simulink model "test_torque"  (R2024b)
settings: Solver=FixedStepDiscrete  StartTime=0.0  StopTime=inf  FixedStep=0.001  RelTol=1e-3
values from neighbouring files (symbols this model uses):
  test_torque_max_nm = 20.0    [test_torque.sldd]
libraries: speedgoatlib_IO614 x4, canmsglib x2
settings Model: DataDictionary=test_torque.sldd  Creator=MFE-HPC  LastModifiedBy=MFE-HPC
settings SolverCC: ConcurrentTasks=on  PositivePriorityOrder=on
settings OptimizationCC: BlockReduction=off  OptimizeBlockIOStorage=off
settings DebuggingCC: TasksWithSamePriorityMsg=none
settings HardwareCC: ProdBitPerLong=64  ProdLongLongMode=on  ProdHWDeviceType=Intel->x86-64 (Linux 64)
settings RTWCC: Description=Speedgoat Real-Time Target Machine  SystemTargetFile=speedgoat.tlc  TemplateMakefile=slrealtime_default_tmf  Toolchain=Simulink Real-Time Toolchain  BuildConfiguration=Faster Runs  CodeExecutionProfiling=on  TargetLang=C++
settings SimulinkRealTimeTargetCC: InstructionSetFMA=off  LogToMDFFile=off

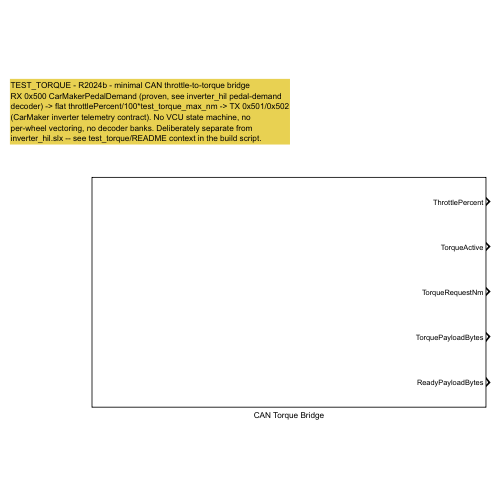
[thumbnail: Simulink's stored preview of the top-level diagram]
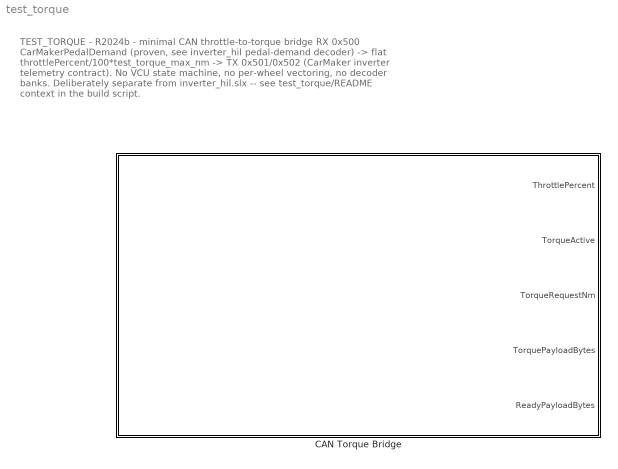
== system test_torque ==
  note: TEST_TORQUE - R2024b - minimal CAN throttle-to-torque bridge
      | RX 0x500 CarMakerPedalDemand (proven, see inverter_hil pedal-demand
      | decoder) -> flat throttlePercent/100*test_torque_max_nm -> TX 0x501/0x502
      | (CarMaker inverter telemetry contract). No VCU state machine, no
      | per-wheel vectoring, no decoder banks. Deliberately separate from
      | inverter_hil.slx -- see test_torque/README context in the build script.
  CAN Torque Bridge : Subsystem

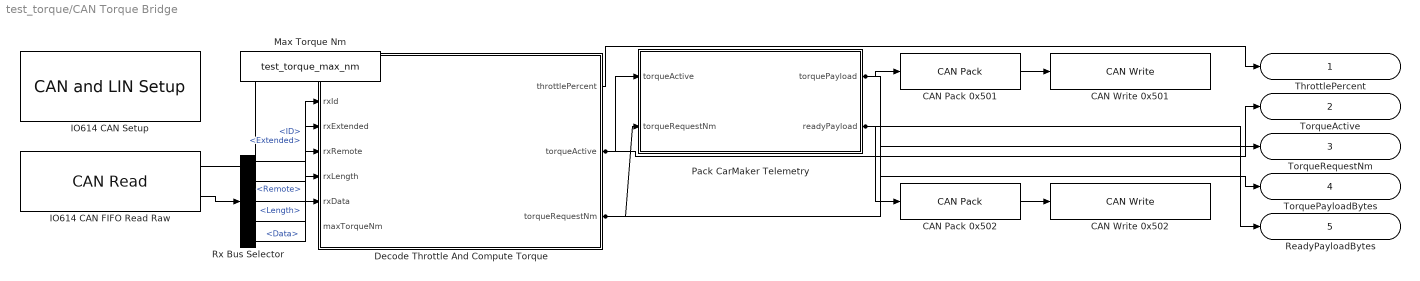
== system test_torque/CAN Torque Bridge ==
  CAN Pack 0x501 : canmsglib/CAN Pack  Description=Torque payload, CarMaker inverter telemetry ID 0x501  MsgList=(none)  MsgName=CAN Msg  MsgIDType=Standard (11-bit identifier)  MsgIdentifier=1281  CANIDInput=off  MsgLength=8  Remote=off  ApplyMinMax=off  BusOutput=off  SignalInfo={}
      settings: LibrarySourceBlock=canlib/CAN Pack  DataFormat=raw data
  CAN Pack 0x502 : canmsglib/CAN Pack  Description=Ready payload, CarMaker inverter telemetry ID 0x502  MsgList=(none)  MsgName=CAN Msg  MsgIDType=Standard (11-bit identifier)  MsgIdentifier=1282  CANIDInput=off  MsgLength=8  Remote=off  ApplyMinMax=off  BusOutput=off  SignalInfo={}
      settings: LibrarySourceBlock=canlib/CAN Pack  DataFormat=raw data
  CAN Write 0x501 : speedgoatlib_IO614/CAN Write   Description=Transmits CarMaker telemetry ID 0x501  moduleType=IO614  id=1  channel=1  canType=CAN (HS)  useBusIn=off  numOfMsg=1  enableInput=off  enableStatusPort=on  initValues=[614 1 0.001 0 1 1 1 1 0 0]  ts=0.001
  CAN Write 0x502 : speedgoatlib_IO614/CAN Write   Description=Transmits CarMaker telemetry ID 0x502  moduleType=IO614  id=1  channel=1  canType=CAN (HS)  useBusIn=off  numOfMsg=1  enableInput=off  enableStatusPort=on  initValues=[614 1 0.001 0 1 1 1 1 0 0]  ts=0.001
  Decode Throttle And Compute Torque : MATLAB Function  TreatAsAtomicUnit=on
  IO614 CAN FIFO Read Raw : speedgoatlib_IO614/CAN Read   moduleType=IO614  id=1  channel=1  canType=CAN (HS)  useBusOut=on  HasMulRead=Single Read from Buffer (FIFO)  MsgIDlist=[1 2]  isEFF=off  LabelInHex=on  enableInput=off  ts=0.001  initValues=[614 1 0.001 0 1 1 0 1 0 1 2 1 2]
  IO614 CAN Setup : speedgoatlib_IO614/CAN and LIN Setup   moduleInitValues="[614    1    1   -1   -1]"  id=1  moduleType=IO614  pciSlot=-1  canChn1=CAN (HS)  canChn2=Disabled  canChn3=Disabled  canChn4=Disabled  linChn1=Disabled  linChn2=Disabled  canInitStructArray=[]  canTermStructArray=[]  canChn1InitValues="[2   2   1  31   8   2   1   5   2]"  arbBdrChn1=1.0 MBaud  arbManBdrChn1=[2,1,31,8]  fdBdrChn1=5.0 MBaud  fdManBdrChn1=[2,1,5,2]  canChn2InitValues="[1   2   1  31   8   2   1   5   2]"  arbBdrChn2=1.0 MBaud  arbManBdrChn2=[2,1,31,8]  fdBdrChn2=5.0 MBaud  fdManBdrChn2=[2,1,5,2]  canChn3InitValues="[1   2   1  31   8   2   1   5   2]"  arbBdrChn3=1.0 MBaud  arbManBdrChn3=[2,1,31,8]  fdBdrChn3=5.0 MBaud  fdManBdrChn3=[2,1,5,2]  canChn4InitValues="[1   2   1  31   8   2   1   5   2]"  arbBdrChn4=1.0 MBaud  arbManBdrChn4=[2,1,31,8]  fdBdrChn4=5.0 MBaud  fdManBdrChn4=[2,1,5,2]  bdrLIN1=19200  linChn1InitValues="[1  19200]"  bdrLIN2=19200  linChn2InitValues="[1  19200]"
      settings: LibrarySourceBlock=speedgoatlib_CANLIN_OfA2/CAN and LIN Setup
  Max Torque Nm : Constant  Value=test_torque_max_nm  SampleTime=0.001
  Pack CarMaker Telemetry : MATLAB Function  TreatAsAtomicUnit=on
  Rx Bus Selector : BusSelector  OutputSignals=ID,Extended,Remote,Length,Data
  ThrottlePercent : Outport
  TorqueActive : Outport  Port=2
  TorqueRequestNm : Outport  Port=3
  TorquePayloadBytes : Outport  Port=4
  ReadyPayloadBytes : Outport  Port=5
  wires:
  ? -> ?
  IO614 CAN FIFO Read Raw/2 -> Rx Bus Selector/1
  IO614 CAN FIFO Read Raw/1 -> Decode Throttle And Compute Torque/1(rxDataPresent)
  Rx Bus Selector/1 -> Decode Throttle And Compute Torque/2(rxId)  "<ID>"
  Rx Bus Selector/2 -> Decode Throttle And Compute Torque/3(rxExtended)  "<Extended>"
  Rx Bus Selector/3 -> Decode Throttle And Compute Torque/4(rxRemote)  "<Remote>"
  Rx Bus Selector/4 -> Decode Throttle And Compute Torque/5(rxLength)  "<Length>"
  Rx Bus Selector/5 -> Decode Throttle And Compute Torque/6(rxData)  "<Data>"
  Max Torque Nm/1 -> Decode Throttle And Compute Torque/7(maxTorqueNm)
  Decode Throttle And Compute Torque/2(torqueActive) -> Pack CarMaker Telemetry/1(torqueActive), TorqueActive/1
  Decode Throttle And Compute Torque/3(torqueRequestNm) -> Pack CarMaker Telemetry/2(torqueRequestNm), TorqueRequestNm/1
  Pack CarMaker Telemetry/1(torquePayload) -> CAN Pack 0x501/1, TorquePayloadBytes/1
  CAN Pack 0x501/1 -> CAN Write 0x501/1
  Pack CarMaker Telemetry/2(readyPayload) -> CAN Pack 0x502/1, ReadyPayloadBytes/1
  CAN Pack 0x502/1 -> CAN Write 0x502/1
  Decode Throttle And Compute Torque/1(throttlePercent) -> ThrottlePercent/1

== matlab function test_torque/CAN Torque Bridge/Pack CarMaker Telemetry ==
  data: torqueActive input; torquePayload output; torqueRequestNm input; readyPayload output
function [torquePayload, readyPayload] = testTorquePackStep( ...
    torqueActive, torqueRequestNm)
%#codegen
%TESTTORQUEPACKSTEP Pack the CarMaker inverter-telemetry pair
%(0x501/0x502) CarMaker's IO.c already decodes into
%MFE_CAN.TorqueRequestTotalNm / MFE_CAN.DriveActive. The entire
%scalar torque request goes in channel 1 (channels 2-4 zero) so the
%C-side four-way sum equals this model's single scalar exactly; the
%ownership gate is broadcast to all four ready bits so the C-side
%four-way OR reduces to the same single gate.
telemetry.torqueSetpointNm = [torqueRequestNm 0 0 0];
telemetry.ready = logical([torqueActive torqueActive torqueActive torqueActive]);
[torquePayload, readyPayload] = inverterhil.packCarMakerTelemetry(telemetry);
end

== matlab function test_torque/CAN Torque Bridge/Decode Throttle And Compute Torque ==
  data: rxDataPresent input; throttlePercent output; rxId input; rxExtended input; rxRemote input; rxLength input; rxData input; maxTorqueNm input; torqueActive output; torqueRequestNm output
function [throttlePercent, torqueActive, torqueRequestNm] = ...
    testTorqueDecodeStep(rxDataPresent, rxId, rxExtended, rxRemote, ...
    rxLength, rxData, maxTorqueNm)
%#codegen
%TESTTORQUEDECODESTEP Decode CarMakerPedalDemand (CAN 0x500) with the
%same hardware-proven CRC-8/SAE-J1850 + alive-counter + 100ms
%freshness logic inverter_hil.slx uses (inverterhil.*), then apply a
%flat linear throttle-percent-to-torque mapping. No PID, no
%per-wheel vectoring, no VCU state machine: torqueRequestNm is zero
%unless CAN pedal ownership is currently held (fresh frame, CRC ok,
%alive counter advanced, Active=1).
persistent bank tickMs
if isempty(bank)
    bank = inverterhil.initialPedalDemandBank();
    tickMs = uint32(0);
end
payload = uint8(rxData(:))';
frame = struct( ...
    'id', uint32(rxId), ...
    'dlc', uint8(rxLength), ...
    'payload', payload, ...
    'isExtended', logical(rxExtended), ...
    'isRemote', logical(rxRemote), ...
    'drop', ~logical(rxDataPresent));
bank = inverterhil.receivePedalDemandFrame(bank, frame, tickMs);
snapshot = inverterhil.pedalDemandSnapshot(bank, tickMs);
throttlePercent = snapshot.throttlePercent;
torqueActive = double(snapshot.ownsPedals);
torqueRequestNm = torqueActive * (throttlePercent / 100) * maxTorqueNm;
tickMs = tickMs + uint32(1);
end
